simulink model "SystemArch"  (R2025a)
settings: Solver=VariableStepAuto  StartTime=0.0  StopTime=10.0  RelTol=1e-3
undefined symbols (not defined in the file): BMS, Camera, Digital, GPS, I2C, IMU, Trhemocouple, UART, UBS1, UBS2, USB1
(part 2 of 2)

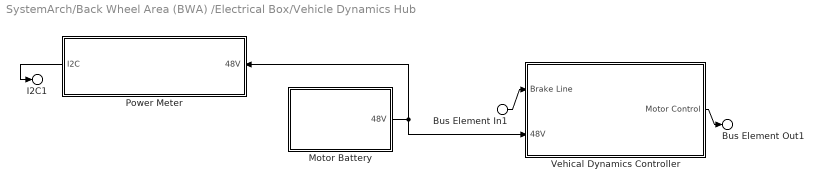
== system SystemArch/Back Wheel Area (BWA) /Electrical Box/Vehicle Dynamics Hub ==
  Bus Element In1 : Inport  PortName=Brake Line
  " Motor Battery" : Subsystem
      settings: PortSchema="{\"entries\":[{\"content\":{\"headerSize\":26,\"margin\":15,\"minimumSpacing\":25,\"sides\":[{\"content\":{},\"type\":\"ConnectorPlacement.EquallySpacedRectSide\",\"uuid\":\"e53759f5-b690-4877-b44a-d4eac11dffdb\"},{\"content\":{\"connectorIds\":[\"Out1\"],\"side\":\"RIGHT\"},\"type\":\"ConnectorPlacement.EquallySpacedRectSide\",\"uuid\":\"5814382e-6b7a-453f-be59-81d6220d088b\"},{\"content\":{\"side\":\"TOP\"},\"type\":\"ConnectorPlacement.EquallySpacedRectSide\",\"uuid\":\"b6b1eca2-b862-4844-b743-dac7054e5132\"}]},\"type\":\"ConnectorPlacement.EquallySpacedConnector\",\"uuid\":\"c2feee16-aff2-42ba-93bb-380b1af0aee9\"}],\"packageUris\":[\"http://schema.mathworks.com/mf0/Connector/R2020b\"],\"version\":\"1.0\"}"
  Power Meter : Subsystem
      settings: PortSchema="{\"entries\":[{\"content\":{\"headerSize\":26,\"margin\":15,\"minimumSpacing\":25,\"sides\":[{\"content\":{\"connectorIds\":[\"Out1\"]},\"type\":\"ConnectorPlacement.EquallySpacedRectSide\",\"uuid\":\"e53759f5-b690-4877-b44a-d4eac11dffdb\"},{\"content\":{\"connectorIds\":[\"In1\"],\"side\":\"RIGHT\"},\"type\":\"ConnectorPlacement.EquallySpacedRectSide\",\"uuid\":\"5814382e-6b7a-453f-be59-81d6220d088b\"},{\"content\":{\"side\":\"TOP\"},\"type\":\"ConnectorPlacement.EquallySpacedRectSide\",\"uuid\":\"b6b1eca2-b862-4844-b743-dac7054e5132\"}]},\"type\":\"ConnectorPlacement.EquallySpacedConnector\",\"uuid\":\"c2feee16-aff2-42ba-93bb-380b1af0aee9\"}],\"packageUris\":[\"http://schema.mathworks.com/mf0/Connector/R2020b\"],\"version\":\"1.0\"}"
  Vehical Dynamics Controller : Subsystem
      settings: PortSchema="{\"entries\":[{\"content\":{\"headerSize\":26,\"margin\":15,\"minimumSpacing\":25,\"sides\":[{\"content\":{\"connectorIds\":[\"In1\",\"In2\"]},\"type\":\"ConnectorPlacement.EquallySpacedRectSide\",\"uuid\":\"b908bc96-20ac-41af-bd35-1dc4c5c5d227\"},{\"content\":{\"connectorIds\":[\"Out1\"],\"side\":\"RIGHT\"},\"type\":\"ConnectorPlacement.EquallySpacedRectSide\",\"uuid\":\"a58e5db6-c2cf-479b-8575-444173ed86e1\"},{\"content\":{\"side\":\"TOP\"},\"type\":\"ConnectorPlacement.EquallySpacedRectSide\",\"uuid\":\"d8b1b400-2606-4583-b904-435fd1d8de03\"},{\"content\":{\"side\":\"BOTTOM\"},\"type\":\"ConnectorPlacement.EquallySpacedRectSide\",\"uuid\":\"f436d6bc-9b26-4b79-a02b-a26636eccfc2\"}]},\"type\":\"ConnectorPlacement.EquallySpacedConnector\",\"uuid\":\"bef962c1-e5c2-4b6f-9336-41c558e2844c\"}],\"packageUris\":[\"http://schema.mathworks.com/mf0/Connector/R2020b\"],\"version\":\"1.0\"}"
  Bus Element Out1 : Outport  PortName=Motor Control
  I2C1 : Outport  Port=2  PortName=I2C
  wires:
  " Motor Battery"/1(48V) -> Power Meter/1(48V), Vehical Dynamics Controller/2(48V)
  Power Meter/1(I2C) -> I2C1/1
  Vehical Dynamics Controller/1(Motor Control) -> Bus Element Out1/1
  Bus Element In1/1 -> Vehical Dynamics Controller/1(Brake Line)

== system SystemArch/Back Wheel Area (BWA) /Rear Wheel/Motor ==
  Bus Element In1 : Inport  PortName=Motor Control

== system SystemArch/Back Wheel Area (BWA) /Electrical Box/Aux. BMS Power Distrubition/Aux Battery ==
  Conn1 : PMIOPort  Side=Right
  Bus Element Out1 : Outport  PortName=5V Raw

== system SystemArch/Back Wheel Area (BWA) /Electrical Box/Aux. BMS Power Distrubition/E-Stop ==
  Bus Element In1 : Inport  PortName=FuseProtected 5V
  Bus Element Out1 : Outport  PortName=E-Stop 5V

== system SystemArch/Back Wheel Area (BWA) /Electrical Box/Aux. BMS Power Distrubition/Fuse ==
  Bus Element In1 : Inport  PortName=5V Raw
  Bus Element Out1 : Outport  PortName=FuseProtected 5V
  wires:
  Bus Element In1/1 -> Bus Element Out1/1

== system SystemArch/Back Wheel Area (BWA) /Electrical Box/Aux. BMS Power Distrubition/Power Meter ==
  Bus Element In1 : Inport  PortName=E-Stop 5V
  Bus Element Out1 : Outport  PortName=5V

== system SystemArch/Back Wheel Area (BWA) /Electrical Box/Aux. BMS Power Distrubition/Thermocouple ==
  Bus Element In1 : Inport  PortName=5V
  Conn1 : PMIOPort  Side=Right
  Bus Element Out1 : Outport  PortName=Trhemocouple[BMS-Digital]

== system SystemArch/Back Wheel Area (BWA) /Electrical Box/Telemetry and Peripherals System/9 Axis IMU ==
  Bus Element In1 : Inport  PortName=5V
  Bus Element Out1 : Outport  PortName=IMU [I2C]

== system SystemArch/Back Wheel Area (BWA) /Electrical Box/Telemetry and Peripherals System/Botton Suite ==
  Bus Element In1 : Inport  PortName=5V
  Bus Element Out1 : Outport  PortName=on/off

== system SystemArch/Back Wheel Area (BWA) /Electrical Box/Telemetry and Peripherals System/GPS ==
  Bus Element In1 : Inport  PortName=5V
  Bus Element Out1 : Outport  PortName=GPS [UART]

== system SystemArch/Back Wheel Area (BWA) /Electrical Box/Telemetry and Peripherals System/Horn ==
  Bus Element In1 : Inport  PortName=on/off

== system SystemArch/Back Wheel Area (BWA) /Electrical Box/Telemetry and Peripherals System/Hotspot ==
  Bus Element Out1 : Outport  PortName=Hotspot [Ethernet port]

== system SystemArch/Back Wheel Area (BWA) /Electrical Box/Telemetry and Peripherals System/LED ==
  Bus Element In1 : Inport  PortName=5V
  Bus Element Out1 : Outport  PortName=LED [PWM]

== system SystemArch/Back Wheel Area (BWA) /Electrical Box/Telemetry and Peripherals System/Light  ==
  Bus Element In1 : Inport  PortName=on/off

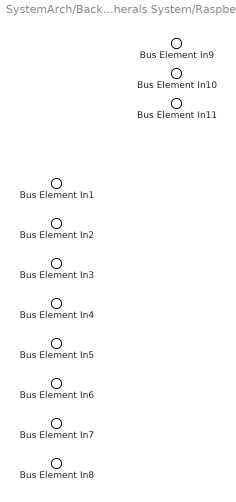
== system SystemArch/Back Wheel Area (BWA) /Electrical Box/Telemetry and Peripherals System/Raspberry Pi ==
  Bus Element In11 : Inport  PortName=Turn Signal
  Bus Element In10 : Inport  Port=2  PortName="Wattes  vlaues"
  Bus Element In9 : Inport  Port=3  PortName=Trhemocouple[BMS-Digital]
  Bus Element In1 : Inport  Port=4  PortName=5V
  Bus Element In2 : Inport  Port=5  PortName=GPS[UART]
  Bus Element In3 : Inport  Port=6  PortName=LED [PWM]
  Bus Element In4 : Inport  Port=7  PortName=IMU[I2C]
  Bus Element In5 : Inport  Port=8  PortName=Camera[UBS1]
  Bus Element In6 : Inport  Port=9  PortName=Camera[UBS2]
  Bus Element In7 : Inport  Port=10  PortName=Hotspot [Ethernet port]
  Bus Element In8 : Inport  Port=11  PortName=I2C

== system SystemArch/Back Wheel Area (BWA) /Electrical Box/Telemetry and Peripherals System/camera (front) ==
  Bus Element In1 : Inport  PortName=5V
  Bus Element Out1 : Outport  PortName=Camera[USB1]

== system SystemArch/Back Wheel Area (BWA) /Electrical Box/Telemetry and Peripherals System/camera (rear) ==
  Bus Element In1 : Inport  PortName=5V
  Bus Element Out1 : Outport  PortName=Camera[UBS2]

== system SystemArch/Back Wheel Area (BWA) /Electrical Box/Vehicle Dynamics Hub/ Motor Battery ==
  Bus Element Out1 : Outport  PortName=48V

== system SystemArch/Back Wheel Area (BWA) /Electrical Box/Vehicle Dynamics Hub/Power Meter ==
  Bus Element In2 : Inport  PortName=48V
  Bus Element Out1 : Outport  PortName=I2C

== system SystemArch/Back Wheel Area (BWA) /Electrical Box/Vehicle Dynamics Hub/Vehical Dynamics Controller ==
  Bus Element In4 : Inport  PortName=Brake Line
  Bus Element In3 : Inport  Port=2  PortName=48V
  Bus Element Out1 : Outport  PortName=Motor Control
